simulink model "full_model_validation_simulation_2015"  (R2020a)
settings: Solver=ode45  StartTime=0.0  StopTime=40  RelTol=1e-3
undefined symbols (not defined in the file): Afe, g, gain_stab9, gains_increasing, I_eq_increasing, K, Kp_i_increasing, Kp_mf_increasing, L, m, m0, Ti_i_increasing, Ti_mf_increasing, x, x_eq, x_eq_increasing, y
libraries: simulink x7
settings Model: Creator=user  LastModifiedBy=miche
settings OptimizationCC: LifeSpan=inf
settings DebuggingCC: IgnoredZcDiagnostic=none  SFExecutionAtInitializationDiag=none  ArithmeticOperatorsInVariantConditions=warning
settings HardwareCC: ProdBitPerSizeT=32  ProdBitPerPtrDiffT=32  ProdWordSize=32  ProdHWDeviceType=Specified
settings SFSimCC: CustomCodeUndefinedFunction=UseInterfaceOnly
settings CodeAppCC: StateflowObjectComments=on

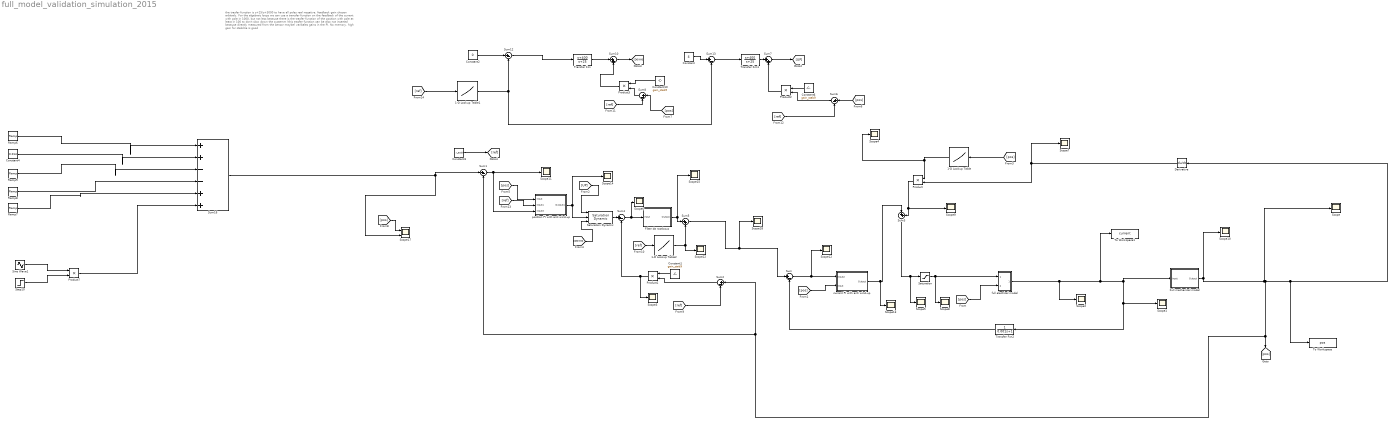
== system full_model_validation_simulation_2015 ==
  note: the trasfer function is s+25/s+3000 to have all poles real negative.
      | feedback gain chosen arbitraly.  For the algebraic loops we can use a transfer function on the feedback of the current with pole in 1000, but not less because there is the trasfer function of the position with pole at least in 100 to don't slow down the systemm (this trasfer function can be also not inserted because directly measured from the sensor maybe)  varibales gains in the PI. No memory. high gain for stabilize is good
  1-D Lookup Table : Lookup_n-D  NumberOfTableDimensions=1  BreakpointsForDimension1=[0.0085 x_eq_increasing]  Table=[gains_increasing(1) gains_increasing]  InternalRulePriority=Speed  RndMeth=Simplest  InputSameDT=on
  1-D Lookup Table1 : Lookup_n-D  NumberOfTableDimensions=1  BreakpointsForDimension1=[0.0085 x_eq_increasing]  Table="[3.55  I_eq_increasing]"  InternalRulePriority=Speed  RndMeth=Simplest  InputSameDT=on
  1-D Lookup Table2 : Lookup_n-D  NumberOfTableDimensions=1  BreakpointsForDimension1=[0.0085 x_eq_increasing]  Table="[3.55  I_eq_increasing]"  InternalRulePriority=Speed  RndMeth=Simplest  InputSameDT=on
  Constant : Constant  Value=4
  Constant1 : Constant  Value=gain_stab9
  Constant10 : Constant  Value=gain_stab9
  Constant2 : Constant  Value=0
  Constant3 : Constant  Value=x_eq(5)
  Constant4 : Constant  Value=0.014
  Constant6 : Constant  Value=gain_stab9
  Derivative : Derivative
  Filter da rootlocus : Subsystem
  Full mechanical model : Subsystem
  Product{,1..3,7} (5 alike) : Product
  Ramp6 : simulink/Sources/Ramp  slope=0.001  start=7  InitialOutput=0
  Ramp7 : simulink/Sources/Ramp  slope=0.001  start=19  InitialOutput=0
  Ramp8 : simulink/Sources/Ramp  slope=0.001  start=17  InitialOutput=0
  Ramp9 : simulink/Sources/Ramp  slope=0.001  start=12  InitialOutput=0
  Saturation : Saturate  UpperLimit=16  LowerLimit=0
  Saturation Dynamic : simulink/Discontinuities/Saturation Dynamic  OutMin=[]  OutMax=[]  OutDataTypeStr=Inherit: Same as second input  OutDataType=fixdt(1, 16)  OutScaling=2^-10  DoSatur=off
  Scope{,1..15,18,22} (18 alike) : Scope
  Scope17 : Scope  NumInputPorts=2
  Sine Wave1 : Sin  Amplitude=0.002  Frequency=3.14  Phase=0.3  SampleTime=0
  Step10 : Step  Time=28  SampleTime=0
  Sum{,1..2,4,6,8,12..13} (8 alike) : Sum  Inputs=|+-
  Sum{3,5,7,10} (4 alike) : Sum  Inputs=|++
  Sum16 : Sum  Inputs=|++--++
  To Workspace : ToWorkspace  VariableName=pos  SampleTime=-1
      settings: Save2DSignal=2-D array (concatenate along first dimension)
  To Workspace1 : ToWorkspace  VariableName=current  SampleTime=-1
      settings: Save2DSignal=2-D array (concatenate along first dimension)
  Transfer Fcn : TransferFcn  Numerator=[1 400]  Denominator=[1 25]
  Transfer Fcn1 : TransferFcn  Numerator=[1 400]  Denominator=[1 25]
  Transfer Fcn2 : TransferFcn  Denominator=[0.001 1]
  current PI with anti wind-up : Subsystem
  full electrical model : Subsystem
  position PI with anti wind-up : Subsystem
  wires:
  [pos] -> 1-D Lookup Table/1
  Sum5/1 -> Scope18/1, Sum/1
  Saturation/1 -> full electrical model/1(In1), Scope8/1
  current PI with anti wind-up/1(Output) -> Scope13/1, Sum3/1
  1-D Lookup Table/1 -> Product/1, Scope4/1
  [pos] -> full electrical model/2(In2)
  Derivative/1 -> Product/2, Scope7/1
  Sum3/1 -> Scope5/1, Saturation/1
  full electrical model/1(Input) -> To Workspace1/1, Full mechanical model/1(Input), Scope1/1, Transfer Fcn2/1, Scope2/1
  [pos] -> current PI with anti wind-up/2(Input)
  Sum/1 -> Scope12/1, current PI with anti wind-up/1(Input2)
  Product/1 -> Scope9/1, Sum3/2
  [UP] -> Saturation Dynamic/1
  Saturation Dynamic/1 -> Sum4/1
  [pos] -> position PI with anti wind-up/1(Input)
  Product1/1 -> Scope3/1, Sum4/2
  [DOWN] -> Saturation Dynamic/3
  Constant1/1 -> Product1/1
  Sum1/1 -> Scope11/1, position PI with anti wind-up/3(Input3)
  Sum2/1 -> Product1/2
  Sum4/1 -> Scope6/1, Filter da rootlocus/1(Input)
  Filter da rootlocus/1(Output) -> Scope15/1, Sum5/1
  [pos] -> Sum8/1
  Sum6/1 -> Product2/2
  Product3/1 -> Sum10/2
  Sum7/1 -> [UP]
  Sum10/1 -> [DOWN]
  Constant6/1 -> Product2/1
  Sum8/1 -> Product3/2
  Transfer Fcn/1 -> Sum10/1
  Transfer Fcn1/1 -> Sum7/1
  Product2/1 -> Sum7/2
  [pos] -> Sum6/1
  Constant10/1 -> Product3/1
  [pos] -> Scope17/1
  [ref] -> 1-D Lookup Table2/1
  [ref] -> position PI with anti wind-up/2(Input1)
  Constant2/1 -> Sum12/1
  [ref] -> 1-D Lookup Table1/1
  Constant/1 -> Sum13/1
  position PI with anti wind-up/1(Output1) -> Saturation Dynamic/2, Scope14/1
  Transfer Fcn2/1 -> Sum/2
  Full mechanical model/1(Output) -> To Workspace/1, Derivative/1, Sum2/1, Sum1/2, [pos], Scope/1, Scope10/1
  1-D Lookup Table2/1 -> Scope22/1, Sum5/2
  [ref] -> Sum2/2
  1-D Lookup Table1/1 -> Sum12/2, Sum13/2
  [ref] -> Sum8/2
  [ref] -> Sum6/2
  Sum13/1 -> Transfer Fcn1/1
  Sum12/1 -> Transfer Fcn/1
  Constant3/1 -> [ref]
  Sine Wave1/1 -> Product7/1
  Ramp8/1 -> Sum16/4
  Ramp7/1 -> Sum16/5
  Product7/1 -> Sum16/6
  Constant4/1 -> Sum16/2
  Ramp6/1 -> Sum16/1
  Step10/1 -> Product7/2
  Ramp9/1 -> Sum16/3
  Sum16/1 -> Scope17/2, Sum1/1

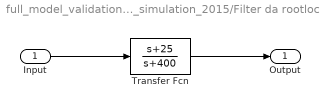
== system full_model_validation_simulation_2015/Filter da rootlocus ==
  Input : Inport
  Transfer Fcn : TransferFcn  Numerator=[1 25]  Denominator=[1 400]
  Output : Outport
  wires:
  Input/1 -> Transfer Fcn/1
  Transfer Fcn/1 -> Output/1

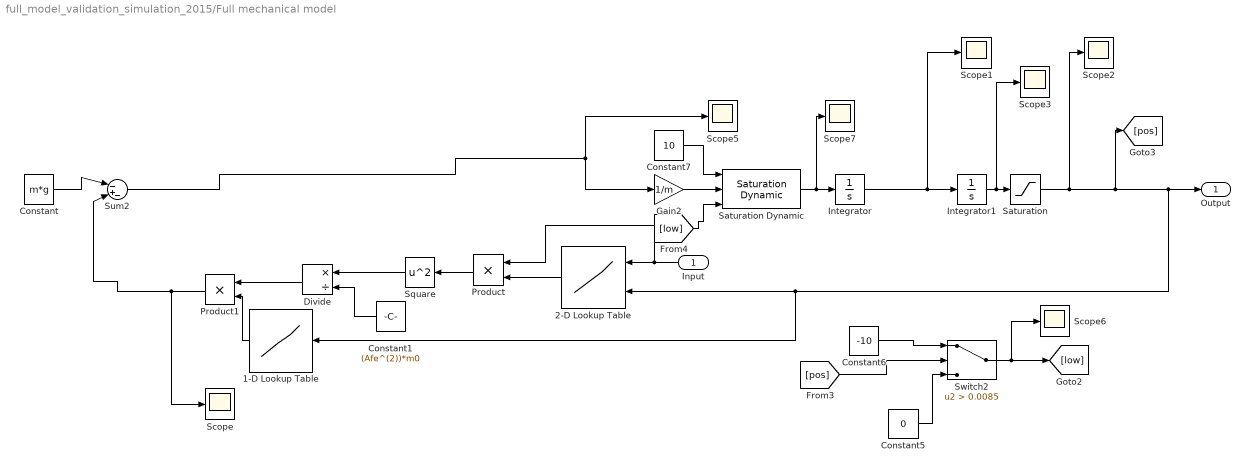
== system full_model_validation_simulation_2015/Full mechanical model ==
  Input : Inport
  1-D Lookup Table : Lookup_n-D  NumberOfTableDimensions=1  BreakpointsForDimension1=x  Table=K  InternalRulePriority=Speed  RndMeth=Simplest  InputSameDT=on
  2-D Lookup Table : Lookup_n-D  BreakpointsForDimension1=y  BreakpointsForDimension2=x  Table=L  InternalRulePriority=Speed  RndMeth=Simplest  InputSameDT=on
  Constant : Constant  Value=m*g
  Constant1 : Constant  Value=(Afe^(2))*m0
  Constant5 : Constant  Value=0
  Constant6 : Constant  Value=-10
  Constant7 : Constant  Value=10
  Divide : Product  Inputs=*/
  Gain2 : Gain  Gain=1/m
  Integrator : Integrator
  Integrator1 : Integrator  InitialCondition=0.0085
  Product : Product
  Product1 : Product
  Saturation : Saturate  UpperLimit=0.020  LowerLimit=0.0085
  Saturation Dynamic : simulink/Discontinuities/Saturation Dynamic  OutMin=[]  OutMax=[]  OutDataTypeStr=Inherit: Same as second input  OutDataType=fixdt(1, 16)  OutScaling=2^-10  DoSatur=off
  Scope{,1..3,5..7} (7 alike) : Scope
  Square : Math  Operator=square  SignedPower=on  SaturateOnIntegerOverflow=on
  Sum2 : Sum  Inputs=|-+-
  Switch2 : Switch  Criteria=u2 > Threshold  Threshold=0.0085
  Output : Outport
  wires:
  Input/1 -> Product/1, 2-D Lookup Table/1
  Square/1 -> Divide/1
  Constant/1 -> Sum2/1
  Product1/1 -> Scope/1, Sum2/2
  Product/1 -> Square/1
  Constant1/1 -> Divide/2
  2-D Lookup Table/1 -> Product/2
  Divide/1 -> Product1/1
  1-D Lookup Table/1 -> Product1/2
  Integrator1/1 -> Scope3/1, Saturation/1
  Integrator/1 -> Scope1/1, Integrator1/1
  Saturation/1 -> Scope2/1, [pos], Output/1, 1-D Lookup Table/1, 2-D Lookup Table/2
  Sum2/1 -> Gain2/1, Scope5/1
  Constant6/1 -> Switch2/1
  [pos] -> Switch2/2
  Switch2/1 -> [low], Scope6/1
  Constant5/1 -> Switch2/3
  Saturation Dynamic/1 -> Scope7/1, Integrator/1
  Gain2/1 -> Saturation Dynamic/2
  [low] -> Saturation Dynamic/3
  Constant7/1 -> Saturation Dynamic/1

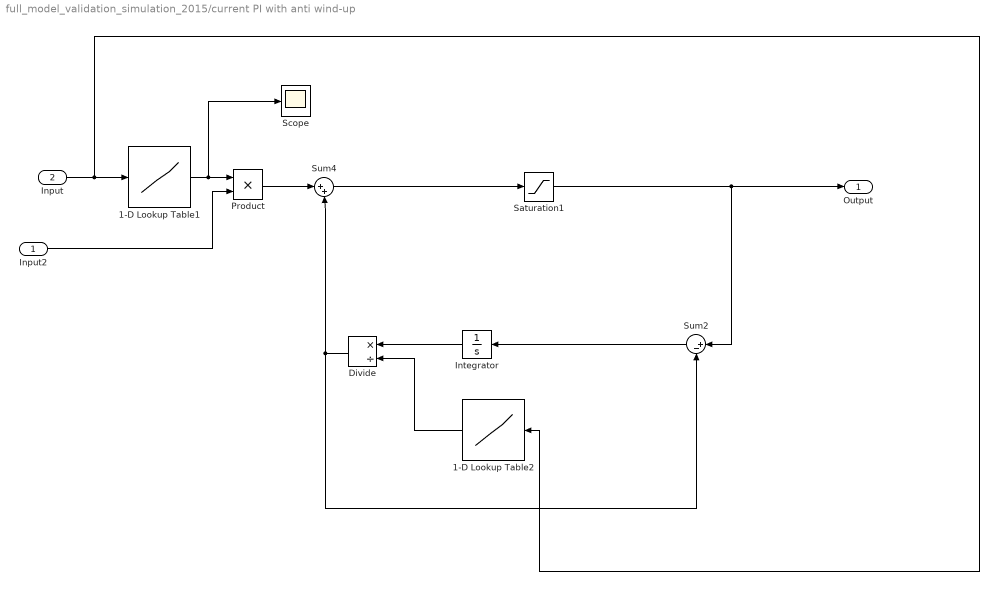
== system full_model_validation_simulation_2015/current PI with anti wind-up ==
  Input2 : Inport
  Input : Inport  Port=2
  1-D Lookup Table1 : Lookup_n-D  NumberOfTableDimensions=1  BreakpointsForDimension1=[0.0085 x_eq_increasing]  Table=[Kp_i_increasing(1) Kp_i_increasing]  InternalRulePriority=Speed  RndMeth=Simplest  InputSameDT=on
  1-D Lookup Table2 : Lookup_n-D  NumberOfTableDimensions=1  BreakpointsForDimension1=[0.0085 x_eq_increasing]  Table=[Ti_i_increasing(1) Ti_i_increasing]  InternalRulePriority=Speed  RndMeth=Simplest  InputSameDT=on
  Divide : Product  Inputs=*/
  Integrator : Integrator
  Product : Product
  Saturation1 : Saturate  UpperLimit=16  LowerLimit=0
  Scope : Scope
  Sum2 : Sum  Inputs=|+-
  Sum4 : Sum  Inputs=|++
  Output : Outport
  wires:
  Sum4/1 -> Saturation1/1
  Product/1 -> Sum4/1
  Saturation1/1 -> Output/1, Sum2/1
  Input2/1 -> Product/2
  1-D Lookup Table1/1 -> Scope/1, Product/1
  Input/1 -> 1-D Lookup Table1/1, 1-D Lookup Table2/1
  Divide/1 -> Sum2/2, Sum4/2
  Sum2/1 -> Integrator/1
  Integrator/1 -> Divide/1
  1-D Lookup Table2/1 -> Divide/2

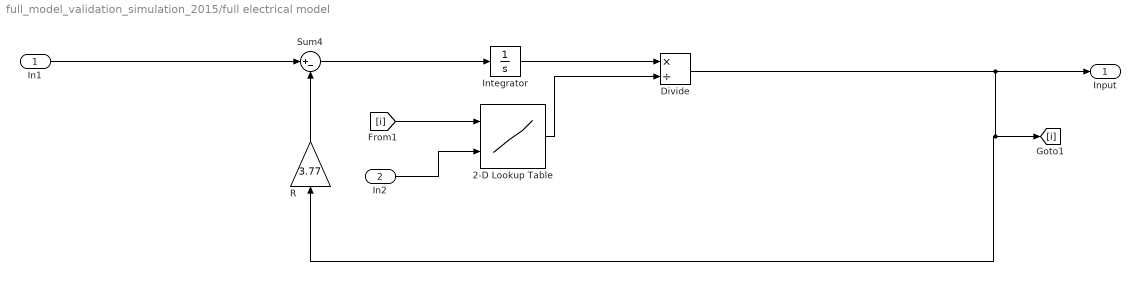
== system full_model_validation_simulation_2015/full electrical model ==
  In1 : Inport
  In2 : Inport  Port=2
  2-D Lookup Table : Lookup_n-D  BreakpointsForDimension1=y  BreakpointsForDimension2=x  Table=L  InternalRulePriority=Speed  RndMeth=Simplest  InputSameDT=on
  Divide : Product  Inputs=*/
  Integrator : Integrator
  R : Gain  Gain=3.77
  Sum4 : Sum  Inputs=|+-
  Input : Outport
  wires:
  Sum4/1 -> Integrator/1
  Integrator/1 -> Divide/1
  R/1 -> Sum4/2
  In2/1 -> 2-D Lookup Table/2
  2-D Lookup Table/1 -> Divide/2
  In1/1 -> Sum4/1
  [i] -> 2-D Lookup Table/1
  Divide/1 -> R/1, [i], Input/1

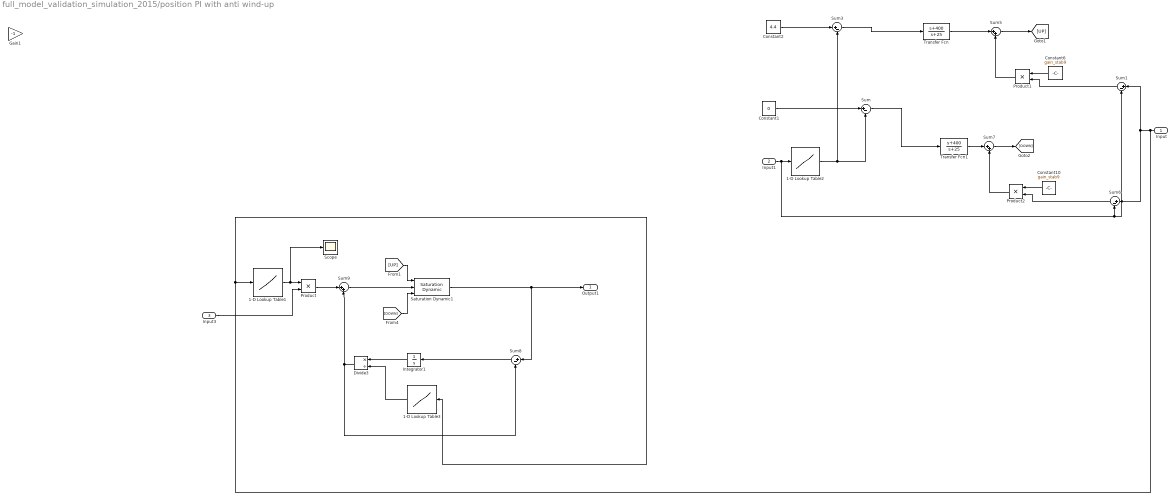
== system full_model_validation_simulation_2015/position PI with anti wind-up ==
  Input : Inport
  Input1 : Inport  Port=2
  Input3 : Inport  Port=3
  1-D Lookup Table1 : Lookup_n-D  NumberOfTableDimensions=1  BreakpointsForDimension1=[0.0085 x_eq_increasing]  Table=[Kp_mf_increasing(1) Kp_mf_increasing]  InternalRulePriority=Speed  RndMeth=Simplest  InputSameDT=on
  1-D Lookup Table2 : Lookup_n-D  NumberOfTableDimensions=1  BreakpointsForDimension1=[0.0085 x_eq_increasing]  Table="[3.55  I_eq_increasing]"  InternalRulePriority=Speed  RndMeth=Simplest  InputSameDT=on
  1-D Lookup Table3 : Lookup_n-D  NumberOfTableDimensions=1  BreakpointsForDimension1=[0.0085 x_eq_increasing]  Table=[Ti_mf_increasing(1) Ti_mf_increasing]  InternalRulePriority=Speed  RndMeth=Simplest  InputSameDT=on
  Constant1 : Constant  Value=0
  Constant10 : Constant  Value=gain_stab9
  Constant2 : Constant  Value=4.4
  Constant6 : Constant  Value=gain_stab9
  Divide3 : Product  Inputs=*/
  Gain1 : Gain  Gain=-1
  Integrator1 : Integrator
  Product : Product
  Product1 : Product
  Product2 : Product
  Saturation Dynamic1 : simulink/Discontinuities/Saturation Dynamic  OutMin=[]  OutMax=[]  OutDataTypeStr=Inherit: Same as second input  OutDataType=fixdt(1, 16)  OutScaling=2^-10  DoSatur=off
  Scope : Scope
  Sum{,1,3,6,8} (5 alike) : Sum  Inputs=|+-
  Sum5 : Sum  Inputs=|++
  Sum7 : Sum  Inputs=|++
  Sum9 : Sum  Inputs=|++
  Transfer Fcn : TransferFcn  Numerator=[1 400]  Denominator=[1 25]
  Transfer Fcn1 : TransferFcn  Numerator=[1 400]  Denominator=[1 25]
  Output1 : Outport
  wires:
  Constant6/1 -> Product1/1
  Sum1/1 -> Product1/2
  Sum7/1 -> [DOWN]
  Product1/1 -> Sum5/2
  Transfer Fcn/1 -> Sum5/1
  Constant10/1 -> Product2/1
  Transfer Fcn1/1 -> Sum7/1
  Sum6/1 -> Product2/2
  Product2/1 -> Sum7/2
  Sum5/1 -> [UP]
  Constant1/1 -> Sum/1
  Constant2/1 -> Sum3/1
  1-D Lookup Table3/1 -> Divide3/2
  Integrator1/1 -> Divide3/1
  Product/1 -> Sum9/1
  Saturation Dynamic1/1 -> Output1/1, Sum8/1
  Input/1 -> 1-D Lookup Table3/1, 1-D Lookup Table1/1, Sum6/1, Sum1/1
  1-D Lookup Table1/1 -> Scope/1, Product/1
  Input3/1 -> Product/2
  Sum9/1 -> Saturation Dynamic1/2
  Sum8/1 -> Integrator1/1
  Divide3/1 -> Sum8/2, Sum9/2
  [UP] -> Saturation Dynamic1/1
  [DOWN] -> Saturation Dynamic1/3
  Input1/1 -> Sum1/2, Sum6/2, 1-D Lookup Table2/1
  1-D Lookup Table2/1 -> Sum/2, Sum3/2
  Sum3/1 -> Transfer Fcn/1
  Sum/1 -> Transfer Fcn1/1
